simulink library "aausat3_lib"  (Simulink 8.3)
settings: Solver=ode45  StartTime=0.0  StopTime=10.0  RelTol=1e-3
undefined symbols (not defined in the file or in its folder): A_wire_mt, albedo_wrapper, alpha_0_mt, bias_gyro, bias_mag, bias_sun, Cd, coil_dim, Dim, f_sample, G, heading_gyro, heading_mag, M_earth, M_moon, M_sun, magnitude, n_mt, noise_gyro, noise_mag, noise_sun, nr_sample_sun, otoquest, otoquest_with_pro, q_method, qmethod, redfac, refldata, s_freq_gyro, s_freq_mag, s_freq_sun, sigma_0_mt, solar_absorb_coeff, solar_m_flux, SVD_method, T_0_mt, theta_e, tilt_gyro, tilt_mag, Ts
undefined symbols (not defined in the file): Actuator_Duty_Cycle_coil, Actuator_Frequency_coil, Dimensions_coil, mean_refl, Number_of_Windings_coil, rho, sim_par, svd_weigth, Wire_Cross_Sectional_Area_coil, Wire_Resistivity_Base_Temperature_coil, Wire_Resistivity_coil, Wire_Resistivity_Temperature_Coefficient_coil
libraries: aausat3_lib x118, simulink_extras x3
(part 1 of 4)
settings Model: Creator=kasperv  LastModifiedBy=Nemanja

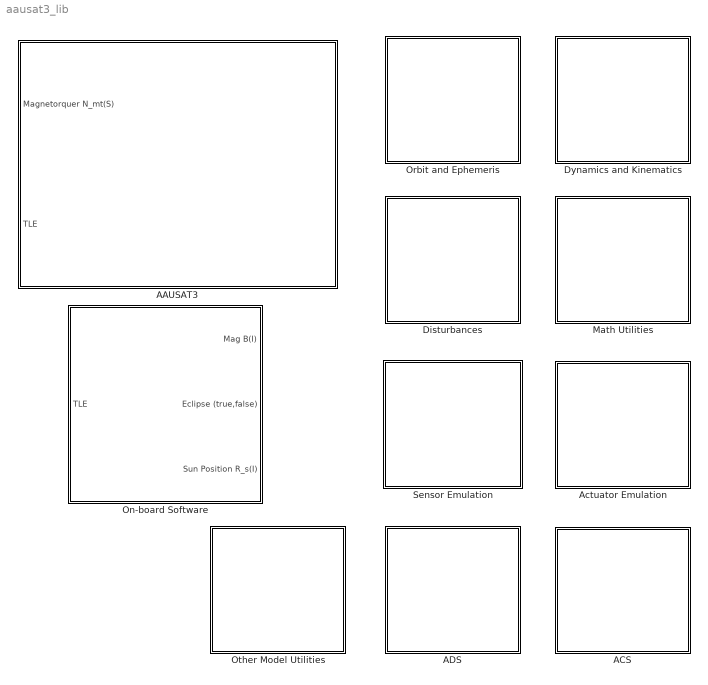
== system aausat3_lib ==
  AAUSAT3 : Subsystem  mask{r_com_s=[0.02 0.001 0.0], sat_temp_start=293.15, mass_sc=2.0, Dim=[0.207 0.1 0.1], inertia_c=[0.007,0.014,0.015], init_jd=2455153.1954318*0, q_s_c=[0 0 0 1], q_init_I_S=[0 1 0 0], w_init_s=[1,1,1]*0.2*(pi/180), Cd=2, rho=0.21850/1e12*0+9.9550/1e12*1+316.2/1e12*0, solar_m_flux=4.5565e-6, solar_absorb_coeff=1.5, theta_e=65, refldata=load('lib/AlbedoToolbox-1.0/refl_data/2005/ga050101-051231'), redfac=1, Ts=1, enable_sensor_emulation=on, enable_env_disturbance=on}
      mask prompts: r_com_s "Center of Mass:"; sat_temp_start "Start Temperature of the Satellite [K]:"; mass_sc "Mass of the Satellite [kg]:"; Dim "Satellite dimension"; inertia_c "Inertia Matrix of the Satellite:"; init_jd "Initial time [JD]:"; q_s_c "Controller Reference Frame (S->C):"; q_init_I_S "Initial Attitude (I->S):"; w_init_s "Initial Angular Rate (S) [rad/s]:"; Cd "Atmospheric Drag Coefficient [-]:"; rho "Atmospheric Density [kg/m^3]:"; solar_m_flux "Solar Momentum Flux [kg/ms^2]:"; solar_absorb_coeff "Solar Absorbtion Coefficient [-]:"; theta_e "Max. Angle of Theta [deg](eclipse: theta>r_earth/norm(R_SA)):"; refldata "Reflectivity Data (REFL Struct):"; redfac "Reduction Factor:"; Ts "Albedo Sampling Time [s]:"; enable_sensor_emulation "Enable Sensor Emulation."; enable_env_disturbance "Enable Environment Disturbance."
      mask Display:
      | image(imread('sat.jpg'));
      | color('w');
      | port_label('input', 1, 'N_mt(S)');
      | port_label('input', 2, 'TLE');
  ACS : Subsystem
      mask Display: image(imread('pictures/control.jpg'))
  ADS : Subsystem
      mask Display: image(imread('pictures/Kalman.jpg'))
  Actuator Emulation : Subsystem
      mask Display: image(imread('pictures/magnetorquer.jpg'))
  Disturbances : Subsystem
      mask Display: image(imread('pictures/noise.jpg'))
  Dynamics and Kinematics : Subsystem
      mask Display: image(imread('pictures/dynamic.jpg'))
  Math Utilities : Subsystem
      mask Display: image(imread('pictures/math.jpg'))
  On-board Software : Subsystem  mask{init_jd=sim_par(20), igrf_order=8, theta_e=65, f_sample=sim_par(22)}
      mask prompts: init_jd "Initial Time [JD]:"; igrf_order "IGRF Model Order [-]:"; theta_e "Max. Angle of Theta [deg]:"; f_sample "Sampling Frequency [Hz]:"
      mask Display:
      | image(imread('pictures/matrix.jpg'));
      | color('w');
      | port_label('input', 1, 'TLE');
      | port_label('output', 1, 'Mag B(I)');
      | port_label('output', 2, 'Eclipse (true,false)');
      | port_label('output', 3, 'Sun Position R_s(I)');
  Orbit and Ephemeris : Subsystem
      mask Display: image(imread('pictures/orbit.jpg'))
  Other Model Utilities : Subsystem
      mask Display: image(imread('pictures/blackboard.jpg'))
  Sensor Emulation : Subsystem
      mask Display: image(imread('pictures/magnetometer.jpg'))

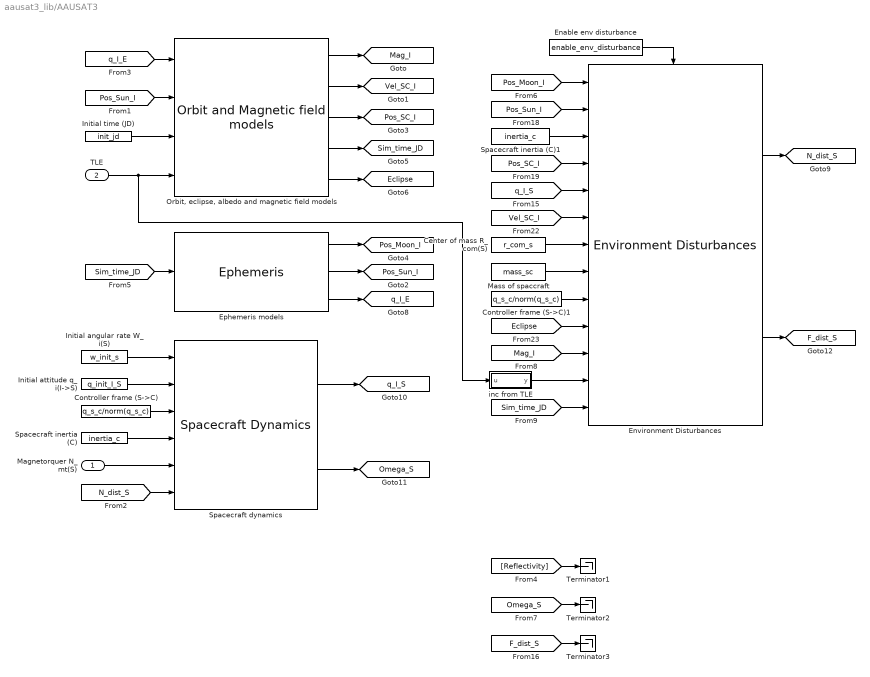
== system aausat3_lib/AAUSAT3 ==
  Magnetorquer N_mt(S) : Inport
  TLE : Inport  Port=2
  Center of mass R_com(S) : Constant  Value=r_com_s
  Controller frame (S->C) : Constant  Value=q_s_c/norm(q_s_c)
  Controller frame (S->C)1 : Constant  Value=q_s_c/norm(q_s_c)
  Enable env disturbance : Constant  Value=enable_env_disturbance
  Environment Disturbances : aausat3_lib/Disturbances/Environment Disturbances  Dim=Dim  sola_m_flux=solar_m_flux  solar_absorb_coeff=solar_absorb_coeff  rho=rho  Cd=Cd  G=6.672e-11  M_sun=1.989e30  M_earth=5.9742e24  M_moon=0.073483e24  enable_rad_dist=on  enable_atmospheric_dist=on  enable_gravity_dist=on  enable_mag_residual_dist=on
  Ephemeris models : aausat3_lib/Orbit and Ephemeris/Ephemeris
  Initial angular rate W_i(S) : Constant  Value=w_init_s
  Initial attitude q_i(I->S) : Constant  Value=q_init_I_S
  Initial time (JD) : Constant  Value=init_jd
  Mass of spaccraft : Constant  Value=mass_sc
  "Orbit, eclipse, albedo and magnetic field models" : aausat3_lib/Orbit and Ephemeris/Orbit and Magnetic field models  theta_e=theta_e  refldata=refldata  redfac=redfac  Ts=Ts  r_e=6371e3  enable_eclipse=on  enable_IGRF=on  reflectivity_enabled=off  enable_sgp4=on  enable_custom_time=on
  Spacecraft dynamics : aausat3_lib/Dynamics and Kinematics/Spacecraft Dynamics
  Spacecraft inertia (C) : Constant  Value=inertia_c
  Spacecraft inertia (C)1 : Constant  Value=inertia_c
  Terminator1 : Terminator
  Terminator2 : Terminator
  Terminator3 : Terminator
  inc from TLE : MATLAB Function  TreatAsAtomicUnit=on
  tag scope: Eclipse=global, F_dist_S=global, Mag_I=global, N_dist_S=global, Omega_S=global, Pos_Moon_I=global, Pos_SC_I=global, Pos_Sun_I=global, Sim_time_JD=global, Vel_SC_I=global, q_I_E=global, q_I_S=global
  wires:
  "Orbit, eclipse, albedo and magnetic field models"/4 -> [Sim_time_JD]
  inc from TLE/1(y) -> Environment Disturbances/12
  [N_dist_S] -> Spacecraft dynamics/6
  [Sim_time_JD] -> Ephemeris models/1
  Spacecraft dynamics/2 -> [Omega_S]
  Ephemeris models/3 -> [q_I_E]
  Ephemeris models/2 -> [Pos_Sun_I]
  Ephemeris models/1 -> [Pos_Moon_I]
  [Sim_time_JD] -> Environment Disturbances/13
  Initial attitude q_i(I->S)/1 -> Spacecraft dynamics/2
  Initial angular rate W_i(S)/1 -> Spacecraft dynamics/1
  "Orbit, eclipse, albedo and magnetic field models"/3 -> [Pos_SC_I]
  Controller frame (S->C)/1 -> Spacecraft dynamics/3
  Spacecraft inertia (C)/1 -> Spacecraft dynamics/4
  "Orbit, eclipse, albedo and magnetic field models"/2 -> [Vel_SC_I]
  "Orbit, eclipse, albedo and magnetic field models"/1 -> [Mag_I]
  Magnetorquer N_mt(S)/1 -> Spacecraft dynamics/5
  "Orbit, eclipse, albedo and magnetic field models"/5 -> [Eclipse]
  [F_dist_S] -> Terminator3/1
  Spacecraft dynamics/1 -> [q_I_S]
  [Pos_Sun_I] -> "Orbit, eclipse, albedo and magnetic field models"/2
  Initial time (JD)/1 -> "Orbit, eclipse, albedo and magnetic field models"/3
  [Reflectivity] -> Terminator1/1
  [Omega_S] -> Terminator2/1
  [q_I_E] -> "Orbit, eclipse, albedo and magnetic field models"/1
  TLE/1 -> "Orbit, eclipse, albedo and magnetic field models"/4, inc from TLE/1(u)
  [Pos_Moon_I] -> Environment Disturbances/1
  Enable env disturbance/1 -> Environment Disturbances/Enable
  [Pos_Sun_I] -> Environment Disturbances/2
  Spacecraft inertia (C)1/1 -> Environment Disturbances/3
  [Pos_SC_I] -> Environment Disturbances/4
  [Vel_SC_I] -> Environment Disturbances/6
  Center of mass R_com(S)/1 -> Environment Disturbances/7
  Mass of spaccraft/1 -> Environment Disturbances/8
  Controller frame (S->C)1/1 -> Environment Disturbances/9
  [Eclipse] -> Environment Disturbances/10
  [Mag_I] -> Environment Disturbances/11
  Environment Disturbances/1 -> [N_dist_S]
  Environment Disturbances/2 -> [F_dist_S]
  [q_I_S] -> Environment Disturbances/5

== system aausat3_lib/ACS ==
  B_dot : Subsystem  mask{C=200000, wc=0.7, m_pm=0.0030, Ts=0.1}
      mask prompts: C "Gain:"; wc "Filter cutoff frequency:"; m_pm "Permanent magnet dipole moment:"; Ts "Sample time:"
  nmpc (AAUSAT3) : Subsystem  mask{f_sample=f_sample}
      mask prompts: f_sample "Sampling Frequency [Hz]"
      mask init:
      | init=0;

== system aausat3_lib/ADS ==
  ADS methods : Subsystem  mask{f_sample=1, svd_weigth=[1/0.0034 1/0.0027], q0_guess=[0 0 1 0], enable_ukf_simple=on, enable_ukf_bias=on, enable_ukf_bias_inertia=off, enable_svd=on}
      mask prompts: f_sample "Sampling Frequency [Hz]:"; svd_weigth "SVD Observations Weights [sun,mag]:"; q0_guess "Initial Attitude Guess [q1,q2,q3,q4]:"; enable_ukf_simple "Enable UKF estimation"; enable_ukf_bias "Enable UKF Plus Bias estimation"; enable_ukf_bias_inertia "Enable UKF Plus Bias and Inertia estimation"; enable_svd "Enable SVD method estimation"
  EKF using quaternions (AAUSAT-II) : Subsystem
  EKF using sun and mag vectors (AAUSAT-II) : Subsystem
  EKF using sun and mag vectors (AAUSAT3) : Subsystem
  EKF using sun and mag vectors ..  and removing bias (AAUSAT-II) : Subsystem
  Propagator from Kalman filter (AAUSAT-II) : Subsystem
  UKF using sun and mag vectors (AAUSAT3) : Subsystem  mask{f_sample=f_sample}
      mask prompts: f_sample "Sampling Frequency [Hz]"
      mask init:
      | init=0;
  UKF using sun and mag vectors .. including bias and inertia estimation (AAUSAT3) : Subsystem  mask{f_sample=f_sample}
      mask prompts: f_sample "Sampling Frequency [Hz]:"
      mask init:
      | init=0;
  UKF using sun and mag vectors .. including bias estimation (AAUSAT3) : Subsystem  mask{f_sample=f_sample}
      mask prompts: f_sample "Sampling Frequency [Hz]:"
      mask init:
      | init=0;
  otoquest (AAUSAT-II) : Subsystem
  otoquest with propagator (AAUSAT-II) : Subsystem
  q-method (AAUSAT-II) : Subsystem
  q-method (AAUSAT3) : Subsystem  mask{weigth_a=[1/(0.031)^2 1/(0.0012)^2]}
      mask prompts: weigth_a "Weigth of the observation vector [-]:"
  svd-method (AAUSAT3) : Subsystem  mask{f_sample=f_sample, weigth_a=svd_weigth}
      mask prompts: f_sample "Sampling Frequency [Hz]:"; weigth_a "Weigth of the Observation Vectors [sun,mag]:"

== system aausat3_lib/Actuator Emulation ==
  Magnetorquer : Subsystem  mask{coil_dim=coil_dim, n_mt=n_mt, A_wire_mt=A_wire_mt, sigma_0_mt=sigma_0_mt, alpha_0_mt=alpha_0_mt, T_0_mt=T_0_mt}
      mask prompts: coil_dim "Coil Dimensions [x,y][m]:"; n_mt "Coil Winding Number [-]:"; A_wire_mt "Wire Cross Sectional Area [m^2]:"; sigma_0_mt "Wire Resistivity [Ohm*m]:"; alpha_0_mt "Wire Resistivity Temperature Coefficient [(deg C)^-1]:"; T_0_mt "Wire Resistivity Base Temperature [K]:"
  Magnetorquers+drivers : Subsystem  mask{coil_dim=Dimensions_coil, n_mt=Number_of_Windings_coil, A_wire_mt=Wire_Cross_Sectional_Area_coil, sigma_0_mt=Wire_Resistivity_coil, alpha_0_mt=Wire_Resistivity_Temperature_Coefficient_coil, T_0_mt=Wire_Resistivity_Base_Temperature_coil, freq_mag=Actuator_Frequency_coil, duty_mag=Actuator_Duty_Cycle_coil}
      mask prompts: coil_dim "Coil Dimensions [x,y][m]:"; n_mt "Coil Winding Number [-]:"; A_wire_mt "Wire Cross Sectional Area [m^2]:"; sigma_0_mt "Wire Resistivity [Ohm*m]:"; alpha_0_mt "Wire Resistivity Temperature Coefficient [(deg C)^-1]:"; T_0_mt "Wire Resistivity Base Temperature [K]:"; freq_mag "Actuator Frequency [Hz]"; duty_mag "Actuator Duty Cycle [%]"
  "Output scaling m -> PWM" : Subsystem  mask{coil_dim=Dimensions_coil, n_mt=Number_of_Windings_coil, A_wire_mt=Wire_Cross_Sectional_Area_coil, sigma_0_mt=Wire_Resistivity_coil, alpha_0_mt=Wire_Resistivity_Temperature_Coefficient_coil, T_0_mt=Wire_Resistivity_Base_Temperature_coil, PWM_max=62.5, PWM_min=37.5}
      mask prompts: coil_dim "Coil Dimensions [x,y][m]:"; n_mt "Coil Winding Number [-]:"; A_wire_mt "Wire Cross Sectional Area [m^2]:"; sigma_0_mt "Wire Resistivity [Ohm*m]:"; alpha_0_mt "Wire Resistivity Temperature Coefficient [(deg C)^-1]:"; T_0_mt "Wire Resistivity Base Temperature [K]:"; PWM_max "PWM max [%]"; PWM_min "PWM min [%]"
  Permanent Magnet : Subsystem  mask{mag_moment=0.0030}
      mask prompts: mag_moment "Magnetic Dipole Moment of the Satellite [Am^2]:"
      mask help: Torque affecting the satellite caused by the magnetic dipole moment.

== system aausat3_lib/Disturbances ==
  Atmospheric : Subsystem  mask{Cd=Cd, rho=rho}
      mask prompts: Cd "Drag Coefficient [-]:"; rho "Atmospheric Density [kg/m^3]:"
      mask help: Force and torque from the atmospheric drag acting on the satellite.
  Environment Disturbances : Subsystem  mask{Dim=Dim, sola_m_flux=solar_m_flux, solar_absorb_coeff=solar_absorb_coeff, rho=rho, Cd=Cd, G=6.672e-11, M_sun=1.989e30, M_earth=5.9742e24, M_moon=0.073483e24, enable_rad_dist=on, enable_atmospheric_dist=on, enable_gravity_dist=on, enable_mag_residual_dist=on}
      mask prompts: Dim "Satellite Dimension [x,y,z][m]:"; sola_m_flux "Solar Momentum Flux [kg/ms^2]:"; solar_absorb_coeff "Solar Absorbtion Coefficient [-]:"; rho "Atmospheric Density [kg/m^3]:"; Cd "Atmospheric Drag Coefficient [-]:"; G "Gravitational Constant [m^3/kgs^2]:"; M_sun "Mass of the Sun [kg]:"; M_earth "Mass of the Earth [kg]:"; M_moon "Mass of the Moon [kg]:"; enable_rad_dist "Enable Radiation Disturbanceses."; enable_atmospheric_dist "Enable Atmospheric Disturbanceses."; enable_gravity_dist "Enable Gravity Disturbanceses."; enable_mag_residual_dist "Enable Magnetic Residual Disturbance"
      mask help: Torque and force from the environment affecting the satellite.
  Gravity : Subsystem  mask{G=G, M_sun=M_sun, M_moon=M_moon, M_earth=M_earth, enable_moon_G=on, enable_sun_G=on, enable_zharm_earth=on, enable_gravity_torque=on}
      mask prompts: G "Gravitational Constant [m^3/kgs^2]:"; M_sun "Mass of the Sun [kg]:"; M_moon "Mass of the Moon [kg]:"; M_earth "Mass of the Earth [kg]:"; enable_moon_G "Enable the Gravity of the Moon."; enable_sun_G "Enable the Gravity of the Sun."; enable_zharm_earth "Enable the Earth Zonal Harmonics."; enable_gravity_torque "Enable Torque From Gravity."
  Gravity Gradient Torque : Subsystem  mask{G=G, M_earth=M_earth}
      mask prompts: G "Gravitational Constant [m^3/kgs^2]:"; M_earth "Mass of the Earth [kg]:"
      mask help: Gravitational force applied by the Earth.
  Gravity Moon : Subsystem  mask{G=G, M_moon=M_moon}
      mask prompts: G "Gravitational Constant [m^3/kgs^2]:"; M_moon "Mass of the Moon [kg]:"
      mask help: Gravitational force applied by the Moon.
  Gravity Sun : Subsystem  mask{G=G, M_sun=M_sun}
      mask prompts: G "Gravitational Constant [m^3/kgs^2]:"; M_sun "Mass of the Sun [kg]:"
      mask help: Gravitational force applied by the Sun.
  Magnetic Residual Disturbance : Subsystem  mask{mag_moment=0.00033}
      mask prompts: mag_moment "Magnetic Dipole Moment of the Satellite [Am^2]:"
      mask help: Torque affecting the satellite caused by the magnetic dipole moment.
  Radiation (I) : Subsystem  mask{Dim=Dim, solar_m_flux=solar_m_flux, solar_absorb_coeff=solar_absorb_coeff}
      mask prompts: Dim "Satellite Dimension [x,y,z][m]:"; solar_m_flux "Solar Momentum Flux [kg/ms^2]:"; solar_absorb_coeff "Absorbtion Coefficient [-]:"
      mask help: Solar force and torque acting on the satellite.
  Zonal Harmonics  Earth : Subsystem

== system aausat3_lib/Dynamics and Kinematics ==
  Spacecraft Dynamics : Subsystem

== system aausat3_lib/Math Utilities ==
  Projection Matrix : Subsystem
  Quaternion operations : Subsystem
  Rotation matrix  to quaternion : MATLABFcn  Description=|  MATLABFcn=A_to_q
      | Converts a rotation matrix to a quaternion.                
      |                                                            
      | The implementation is implemented to be numerically robust.
  Vector operations : Subsystem
  q_i_o calculator : Subsystem

== system aausat3_lib/On-board Software ==
  TLE : Inport
  Constant : Constant  Value=init_jd  SampleTime=1/f_sample
  Ephemeris : Subsystem
  Orbit and Magnetic field models : Subsystem  mask{r_e=6371e3, theta_e=theta_e, init_jd=init_jd, igrf_order=igrf_order, enable_eclipse=on, enable_IGRF=on, enable_sgp4=on, enable_custom_time=on}
      mask prompts: r_e "Radius of the Earth [m]:"; theta_e "Max. Angle of Theta [deg] (eclipse: theta > r_earth/norm(R_SA)):"; init_jd "Initial Time [JD]:"; igrf_order "IGRF Model Order [-]:"; enable_eclipse "Enable Eclipse Model."; enable_IGRF "Enable IGRF Model."; enable_sgp4 "Enable SGP4 Model."; enable_custom_time "Enable Custom Time."
  Mag B(I) : Outport  SampleTime=1/f_sample
  Eclipse (true,false) : Outport  Port=2  SampleTime=1/f_sample
  Sun Position R_s(I) : Outport  Port=3  SampleTime=1/f_sample
  tag scope: Sim_time_JD_sat=global, q_I_E_sat=global
  wires:
  Orbit and Magnetic field models/2(Simulation time t(JD)) -> [Sim_time_JD_sat]
  Orbit and Magnetic field models/3("Eclipse: 1=true, 0=false") -> Eclipse (true,false)/1
  Orbit and Magnetic field models/1(Mag [Tesla] B(I)) -> Mag B(I)/1
  TLE/1 -> Orbit and Magnetic field models/4(TLE)
  [Sim_time_JD_sat] -> Ephemeris/1(Time t(JD))
  [q_I_E_sat] -> Orbit and Magnetic field models/1(Earth rotation q(I->E))
  Ephemeris/1(Sun Position R_s(I)) -> Sun Position R_s(I)/1, Orbit and Magnetic field models/2(Sun position R_s(I))
  Ephemeris/2(Earth Rotation q(I->E)) -> [q_I_E_sat]
  Constant/1 -> Orbit and Magnetic field models/3(Initial time ti(JD))

== system aausat3_lib/Orbit and Ephemeris ==
  (IGRF) Magnetic field : Subsystem  TreatAsAtomicUnit=on
  Albedo : Subsystem  TreatAsAtomicUnit=on  mask{refldata=mean_refl, redfac=1, Ts=-1}
      mask prompts: refldata "Reflectivity Data (REFL Struct):"; redfac "Reduction factor:"; Ts "Sample Time (-1 for inherited):"
  Custom time : Subsystem  TreatAsAtomicUnit=on
  ECI->ECEF quaternion : Subsystem
  Eclipse model : Subsystem  mask{r_e=6371000, enable=off, theta_e=65}
      mask prompts: r_e "Radius of Earth [m]"; enable "Enable max angle"; theta_e "Max. angle of theta [deg] (eclipse: theta > r_earth/norm(R_SA))"
      mask Display: fprintf('1=true,\n 0=false')
  Ephemeris : Subsystem
  Magnetic field model : Subsystem
  Orbit and Magnetic field models : Subsystem  mask{theta_e=theta_e, refldata=refldata, redfac=redfac, Ts=Ts, r_e=6371e3, enable_eclipse=on, enable_IGRF=on, reflectivity_enabled=off, enable_sgp4=on, enable_custom_time=on}
      mask prompts: theta_e "Max. Angle of Theta [deg] (eclipse: theta > r_earth/norm(R_SA)):"; refldata "Reflectivity Data (REFL Struct):"; redfac "Reduction Factor:"; Ts "Albedo Model Sampling Time [s]:"; r_e "Radius of the Earth [m]:"; enable_eclipse "Enable Eclipse Model."; enable_IGRF "Enable IGRF Model."; reflectivity_enabled "Enable Albedo Model."; enable_sgp4 "Enable SGP4 Model."; enable_custom_time "Enable Custom Time."
      mask help: When you want to use "Other" make sure to define the TLE in the SGP4 subsystem.
  SGP4 position : Subsystem  TreatAsAtomicUnit=on
  TLE AAUSAT-II : Subsystem  mask{satname='AAUSAT-II', JulianDay=09279.82913737, xndt2o=0.00000416, xndd6o=0.0, bstar=.59418e-4, xincl=97.9326, xnodeo=342.7215, eo=0.0016322, omegao=34.9001, xmo=325.3249, xno=14.81792083, ts=1}
      mask prompts: satname "Satellite Name:"; JulianDay "Epoch [YYDDD.DDDDDDDD]:"; xndt2o "Mean Motion 1st [rev/day^2]:"; xndd6o "Mean Motion 2nd [rev/day^3]:"; bstar "B* Drag [Earth radii^-1]"; xincl "Inclination [deg]:"; xnodeo "Right Ascension of Ascending Node [deg]:"; eo "Eccentricity [-]:"; omegao "Argument of Perigee [deg]:"; xmo "Mean Anomaly [deg]:"; xno "Mean Motion [rev/day]:"; ts "Sampling Time [sec]:"
      mask help: Two-Line Orbital Element Set Format.
      mask Display: fprintf('TLE Object \n Satellite Name: %s\n Epoch: %d',satname,floor(JulianDay));
  TLE AAUSAT-II (2) : aausat3_lib/Orbit and Ephemeris/TLE AAUSAT-II  satname='AAUSAT-II'  JulianDay=09321.69542252  xndt2o=0.00000555  xndd6o=0.0  bstar=.76898e-4  xincl=97.9251  xnodeo=24.1597  eo=0.0014245  omegao=254.1774  xmo=105.7862  xno=14.81823818  ts=1
  TLE Orsted : Subsystem  mask{satname='Orsted', YYDDD=02039, JulianDay=2452275.5+40.69255057, xndt2o=0.00002748*0, xndd6o=0, bstar=0.00071190, xincl=96.4788, xnodeo=112.1945, eo=0.0148615, omegao=71.6037, xmo=290.1241, xno=14.43891950, ts=1}
      mask prompts: satname "Satellite Name:"; YYDDD "Epoch [YYDDD]:"; JulianDay "Epoch [JD]:"; xndt2o "Mean Motion 1st [rev/day^2]:"; xndd6o "Mean Motion 2nd [rev/day^3]:"; bstar "B* Drag [Earth radii^-1]"; xincl "Inclination [deg]:"; xnodeo "Right Ascension of Ascending Node [deg]:"; eo "Eccentricity [-]:"; omegao "Argument of Perigee [deg]:"; xmo "Mean Anomaly [deg]:"; xno "Mean Motion [rev/day]:"; ts "Sampling Time [sec]:"
      mask help: Two-Line Orbital Element Set Format.
      mask Display: fprintf('TLE Object \n Satellite Name: %s\n Epoch: %d',satname,YYDDD);

== system aausat3_lib/Other Model Utilities ==
  AAUSAT-II Animation : Subsystem  mask(AAUSAT-II Animation){u1=[-20000000 20000000 -20000000 20000000 -20000000 20000000], u2=1, u3=300000, u20=on, u18=15, u4=6378000, u11=150, u12=on, u13='earth3150.jpg', u17=180, u5=Fixed position, u6=[70000000 70000000 70000000], u7=8, u9=off, u10=on, u16=off, u14=on, u15=on, u8=on, u19=off}
      mask prompts: u1 "Axes limits [xmin xmax ymin ymax zmin zmax]:"; u2 "Time interval between updates:"; u3 "Size of spacecraft displayed:"; u20 "Use spacecraft image map"; u18 "Spacecraft drawing slices"; u4 "Planet radius:"; u11 "Planet drawing slices"; u12 "Use planet map"; u13 "Planet map image file"; u17 "Pre-rotate image map (deg)"; u5 "Enter view:"; u6 "Position of camera [xc yc zc]:"; u7 "View angle:"; u9 "Show SC coordinate system"; u10 "Show orbit coordinate system"; u16 "Show Earth Centered Earth Fixed coordinate system"; u14 "Show inertial coordinate system"; u15 "Show trajectory"; u8 "Enable animation"; u19 "Make movie (use with care!)"
      mask help:
      | Create a 3-D animated view of the AAUSAT-II, where X, Y, and Z craft position (Position) and craft quaternion (Attitude) are inputs.
      |
      | Display parameters are in the same units of length as the input parameters.
      |
      | Created by Karl Laursen
      mask init:
      | Config.axes = u1;
      | Config.update = u2;
      | Config.craft = u3;
      | Config.radius = u4;
      | Config.camera_view = u5;
      | Config.camera_pos = u6;
      | Config.view = u7;
      | Config.Animenable = u8;
      | Config.ShowSCFrame = u9;
      | Config.ShowOrbitFrame = u10;
      | Config.ShowECEF = u16;
      | Config.ShowInertial = u14;
      | Config.PlanetSlices = u11;
      | Config.UseMap = u12;
      | Config.PlanetMapFile = u13;
      | Config.Trajectory = u15;
      | Config.PreRotation = u17;
      | Config.CraftSlices = u18;
      | Config.MakeMovie = u19;
      | Config.UseSCMap = u20;
      mask Help: web(asbhelp('6dofanimation'));
      mask TypeOptions u5: Fixed position | Fly alongside
  Exposed area : Subsystem  mask{dim_sat_area=[0.1,0.2,0.1]}
      mask prompts: dim_sat_area "Satellite Dimentions [x,y,z] [m]:"
      mask help: Calculates the exposed area of the satellite.
  Geocentric to  Geodetic Latitude : Subsystem  mask(Geocentric to Geodetic Latitude){F=, R=}
      mask prompts: F "Flattening:"; R "Equatorial radius of planet:"
      mask help: Convert geocentric latitude to geodetic latitude. Geodetic latitude is computed using geocentric latitude and the radius from the center of the planet to the center of gravity.
      mask init:
      | F=1/298.257223563;
      | R=6378137;
      mask Help: eval('asbhelp');
      mask Display:
      | port_label('input',1,'\lambda','texmode','on')
      | port_label('input',2,'r','texmode','on')
      | port_label('output',1,'\mu','texmode','on')
  Geodetic to  Geocentric Latitude : Subsystem  mask(Geodetic to Geocentric Latitude){F=1/298.257223563, R=6378137}
      mask prompts: F "Flattening:"; R "Equatorial radius of planet:"
      mask help: Convert geodetic latitude to geocentric latitude. Setting mean sea-level altitude to zero will give the geocentric latitude at the surface of the planet.
      mask Help: eval('asbhelp');
      mask Display:
      | port_label('input',1,'\mu','texmode','on')
      | port_label('input',2,'h','texmode','on')
      | port_label('output',1,'\lambda','texmode','on')
  Randome 3D Vector : Subsystem  mask{mean=0, var=100, seed=[23314,67594,99812]}
      mask prompts: var "Variance:"; seed "Seed [s1,s2,s3]:"
  SC ECI to geodetic position converter : Subsystem
      mask help:
      | Converts the spacecraft position in the ECI frame to geodetic coordinates.
      | Can be used to plot spacecraft position on a world map.
      mask init:
      | a=6378.1370;
      | b=6356.7523;
  Satellite Area : Subsystem
  Store data : Subsystem  mask{f_sample=1, enable_t=on, enable_att=on, enable_w=on, enable_att_ukf=on, enable_w_ukf=on, enable_r_sun=on, enable_r_mag=on, enable_r_w=on, enable_eia=on, enable_eiw=on, enable_att_ukf_bias=on, enable_w_ukf_bias=on, enable_b_mag=on, enable_b_gyro=on, enable_r_sun_ukf_bias=on, enable_r_mag_ukf_bias=on, enable_r_w_ukf_bias=on, enable_eia_ukf_bias=on, enable_eiw_ukf_bias=on, enable_att_svd=on, enable_svd_att_err=on, enable_svd_err=on, enable_tictoc=on, enable_tictoc_ukf_bias=on, enable_tictoc_svd=on, enable_n_dist=on, enable_n_pmag=on, enable_n_con=on, enable_eclip_sw=on, enable_eclip_real=on}
      mask prompts: f_sample "Sampling Frequency [Hz]:"; enable_t "Store Time"; enable_att "Store Real Attitude"; enable_w "Store Real Angular Velocity"; enable_att_ukf "Store Estimated Attitude (UKF)"; enable_w_ukf "Store Estimated Angular Velocity (UKF)"; enable_r_sun "Store Sun Vector Residual (UKF)"; enable_r_mag "Store Magnetic Field Vector Residual (UKF)"; enable_r_w "Store Angular Velocity Residual (UKF)"; enable_eia "Store Error in Attitude  (UKF)"; enable_eiw "Store Error in Angular Velocity (UKF)"; enable_att_ukf_bias "Store Estimated Attitude (UKF Bias)"; enable_w_ukf_bias "Store Estimated Angular Velocity (UKF Bias)"; enable_b_mag "Store Magnetometer Bias (UKF Bias)"; enable_b_gyro "Store Gyro Bias (UKF Bias)"; enable_r_sun_ukf_bias "Store Sun Vector Residual (UKF Bias)"; enable_r_mag_ukf_bias "Store Magnetic Field Vector Residual (UKF Bias)"; enable_r_w_ukf_bias "Store Angular Velocity Residual (UKF Bias)"; enable_eia_ukf_bias "Store Error in Attitude  (UKF Bias)"; enable_eiw_ukf_bias "Store Error in Angular Velocity (UKF Bias)"; enable_att_svd "Store Estimated Attitude (SVD)"; enable_svd_att_err "Store Error in Attitude (SVD)"; enable_svd_err "Store SVD Error Indicator"; enable_tictoc "Store Algorithm Execution Time (UKF)"; enable_tictoc_ukf_bias "Store Algorithm Execution Time (UKF Bias)"; enable_tictoc_svd "Store Algorithm Execution Time (SVD)"; enable_n_dist "Store Environment Disturbances"; enable_n_pmag "Store Permanent Magnet Disturbance"; enable_n_con "Store Control Torque"; enable_eclip_sw "Stor On-board Software Eclipse Indicator"; enable_eclip_real "Store the Real Eclipse Indicator"
  "TLE -> JD converter" : Subsystem

== system aausat3_lib/Sensor Emulation ==
  Gyroscopes : Subsystem  mask{s_freq_gyro=s_freq_gyro, noise_gyro=noise_gyro, bias_gyro=bias_gyro, heading_gyro=heading_gyro, tilt_gyro=tilt_gyro}
      mask prompts: s_freq_gyro "Sampling Frequency [Hz]:"; noise_gyro "Noise [deg/s]:"; bias_gyro "Bias (x,y,z) [deg/s]:"; heading_gyro "Sensor placement error (heading) [deg]:"; tilt_gyro "Sensor placement error (tilt) [deg]:"
  Magnetometers : Subsystem  mask{s_freq_mag=s_freq_mag, noise_mag=noise_mag, bias_mag=bias_mag, heading_mag=heading_mag, tilt_mag=tilt_mag}
      mask prompts: s_freq_mag "Sampling Frequency [Hz]:"; noise_mag "Noise [deg]:"; bias_mag "Bias (x,y,z) [nT]:"; heading_mag "Sensor placement error (heading) [deg]:"; tilt_mag "Sensor placement error (tilt) [deg]:"
  Measurements : Subsystem  mask{s_freq_mag=1, noise_mag=3, bias_mag=[0 0 0], heading_mag=0, tilt_mag=0, s_freq_sun=1, noise_sun=3.33, bias_sun=[0 0], nr_sample_sun=1, s_freq_gyro=1, noise_gyro=0.2, bias_gyro=[0 0 0], heading_gyro=0, tilt_gyro=0}
      mask prompts: s_freq_mag "Magnetometer Sampling Frequency [Hz]:"; noise_mag "Magnetometer Noise [deg]:"; bias_mag "Magnetometer Bias (x,y,z) [nT]:"; heading_mag "Magnetometer Placement Error (heading) [deg]:"; tilt_mag "Magnetometer Placement Error (tilt) [deg]:"; s_freq_sun "Sun Sensor Sampling Frequency [Hz]:"; noise_sun "Sun Sensor Noise [deg]:"; bias_sun "Sun Sensor Bias (theta,phi) [deg]:"; nr_sample_sun "Number of Sun Samples [-]:"; s_freq_gyro "Gyroscope Sampling Frequency [Hz]:"; noise_gyro "Gyroscope Noise [deg/s]:"; bias_gyro "Gyroscope Bias (x,y,z) [deg/s]:"; heading_gyro "Gyroscope Placement Error (heading) [deg]:"; tilt_gyro "Gyroscope Placement Error (tilt) [deg]:"
  Sun sensors : Subsystem  mask{s_freq_sun=s_freq_sun, noise_sun=noise_sun, bias_sun=bias_sun, nr_sample_sun=nr_sample_sun}
      mask prompts: s_freq_sun "Sampling Frequency [Hz]:"; noise_sun "Noise [deg]:"; bias_sun "Bias (theta,phi) [deg]:"; nr_sample_sun "Number of Samples [-]:"

== system aausat3_lib/ACS/B_dot ==
  B_meas : Inport
  Gain : Gain  Gain=-C
  Gain1 : Gain  Gain=wc
  Gain2 : Gain  Gain=exp(-wc*Ts)
  Permanent magnet  dipole moment : Constant  Value=[0,0,m_pm]
  Sum2 : Sum  Inputs=-++
  Sum3 : Sum  Inputs=|++
  Unit Delay : UnitDelay  SampleTime=-1
  Unit Delay1 : UnitDelay  SampleTime=-1
  m_ctrl : Outport  PortDimensions=3
  wires:
  B_meas/1 -> Gain1/1
  Unit Delay/1 -> Sum2/1
  Gain1/1 -> Unit Delay/1, Sum2/2
  Gain2/1 -> Sum2/3
  Unit Delay1/1 -> Gain2/1
  Sum2/1 -> Unit Delay1/1, Gain/1
  Permanent magnet  dipole moment/1 -> Sum3/2
  Gain/1 -> Sum3/1
  Sum3/1 -> m_ctrl/1

== system aausat3_lib/ACS/nmpc (AAUSAT3) ==
  x0 : Inport
  q_ref : Inport  Port=2
  simtime_JD : Inport  Port=3
  Enable : EnablePort
  Mux2 : Mux  Inputs=3
  UKF : MATLABFcn  MATLABFcn=nmpc  OutputDimensions=3  SampleTime=1/f_sample
  Uctrl : Outport
  wires:
  q_ref/1 -> Mux2/2
  x0/1 -> Mux2/1
  UKF/1 -> Uctrl/1
  Mux2/1 -> UKF/1
  simtime_JD/1 -> Mux2/3

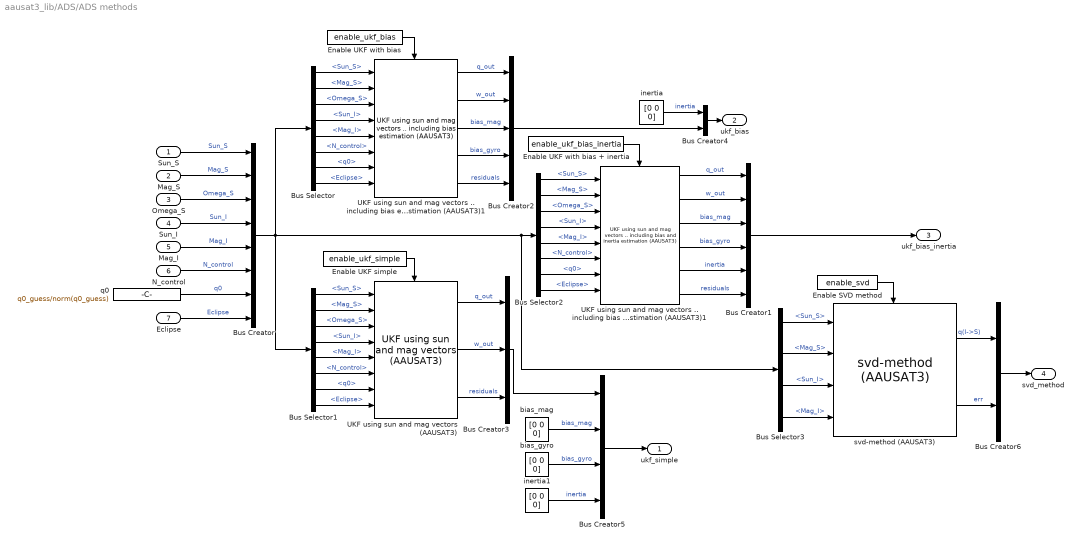
== system aausat3_lib/ADS/ADS methods ==
  Sun_S : Inport
  Mag_S : Inport  Port=2
  Omega_S : Inport  Port=3
  Sun_I : Inport  Port=4
  Mag_I : Inport  Port=5
  N_control : Inport  Port=6
  Eclipse : Inport  Port=7
  Bus Creator : BusCreator  Inputs=8
  Bus Creator1 : BusCreator  Inputs=6
  Bus Creator2 : BusCreator  Inputs=5
  Bus Creator3 : BusCreator  Inputs=3
  Bus Creator4 : BusCreator  Inputs=2
  Bus Creator5 : BusCreator
  Bus Creator6 : BusCreator  Inputs=2
  Bus Selector : BusSelector  OutputSignals=Sun_S,Mag_S,Omega_S,Sun_I,Mag_I,N_control,q0,Eclipse
  Bus Selector1 : BusSelector  OutputSignals=Sun_S,Mag_S,Omega_S,Sun_I,Mag_I,N_control,q0,Eclipse
  Bus Selector2 : BusSelector  OutputSignals=Sun_S,Mag_S,Omega_S,Sun_I,Mag_I,N_control,q0,Eclipse
  Bus Selector3 : BusSelector  OutputSignals=Sun_S,Mag_S,Sun_I,Mag_I
  Enable SVD method : Constant  Value=enable_svd
  Enable UKF simple : Constant  Value=enable_ukf_simple
  Enable UKF with bias : Constant  Value=enable_ukf_bias
  Enable UKF with bias + inertia : Constant  Value=enable_ukf_bias_inertia
  UKF using sun and mag vectors (AAUSAT3) : aausat3_lib/ADS/UKF using sun and mag vectors (AAUSAT3)  SystemSampleTime=-1  f_sample=f_sample
  UKF using sun and mag vectors .. including bias and inertia estimation (AAUSAT3)1 : aausat3_lib/ADS/UKF using sun and mag vectors .. including bias and inertia estimation (AAUSAT3)  SystemSampleTime=-1  f_sample=f_sample
  UKF using sun and mag vectors .. including bias estimation (AAUSAT3)1 : aausat3_lib/ADS/UKF using sun and mag vectors .. including bias estimation (AAUSAT3)  SystemSampleTime=-1  f_sample=f_sample
  bias_gyro : Constant  Value=[0 0 0]
  bias_mag : Constant  Value=[0 0 0]
  inertia : Constant  Value=[0 0 0]
  inertia1 : Constant  Value=[0 0 0]
  q0 : Constant  Value=q0_guess/norm(q0_guess)
  svd-method (AAUSAT3) : aausat3_lib/ADS/svd-method (AAUSAT3)  SystemSampleTime=-1  f_sample=f_sample  weigth_a=svd_weigth
  ukf_simple : Outport
  ukf_bias : Outport  Port=2
  ukf_bias_inertia : Outport  Port=3
  svd_method : Outport  Port=4
  wires:
  Bus Creator6/1 -> svd_method/1
  svd-method (AAUSAT3)/2 -> Bus Creator6/2  "err"
  svd-method (AAUSAT3)/1 -> Bus Creator6/1  "q(I->S)"
  Bus Creator/1 -> Bus Selector/1, Bus Selector1/1, Bus Selector3/1, Bus Selector2/1
  Bus Creator5/1 -> ukf_simple/1
  inertia1/1 -> Bus Creator5/4  "inertia"
  bias_gyro/1 -> Bus Creator5/3  "bias_gyro"
  bias_mag/1 -> Bus Creator5/2  "bias_mag"
  Bus Creator3/1 -> Bus Creator5/1
  Bus Creator4/1 -> ukf_bias/1
  Bus Creator2/1 -> Bus Creator4/2
  inertia/1 -> Bus Creator4/1  "inertia"
  Sun_S/1 -> Bus Creator/1  "Sun_S"
  Mag_S/1 -> Bus Creator/2  "Mag_S"
  Omega_S/1 -> Bus Creator/3  "Omega_S"
  Sun_I/1 -> Bus Creator/4  "Sun_I"
  Mag_I/1 -> Bus Creator/5  "Mag_I"
  N_control/1 -> Bus Creator/6  "N_control"
  q0/1 -> Bus Creator/7  "q0"
  Eclipse/1 -> Bus Creator/8  "Eclipse"
  Bus Selector/1 -> UKF using sun and mag vectors .. including bias estimation (AAUSAT3)1/1  "<Sun_S>"
  Bus Selector/2 -> UKF using sun and mag vectors .. including bias estimation (AAUSAT3)1/2  "<Mag_S>"
  Bus Selector/3 -> UKF using sun and mag vectors .. including bias estimation (AAUSAT3)1/3  "<Omega_S>"
  Bus Selector/4 -> UKF using sun and mag vectors .. including bias estimation (AAUSAT3)1/4  "<Sun_I>"
  Bus Selector/5 -> UKF using sun and mag vectors .. including bias estimation (AAUSAT3)1/5  "<Mag_I>"
  Bus Selector/6 -> UKF using sun and mag vectors .. including bias estimation (AAUSAT3)1/6  "<N_control>"
  Bus Selector/7 -> UKF using sun and mag vectors .. including bias estimation (AAUSAT3)1/7  "<q0>"
  Bus Selector/8 -> UKF using sun and mag vectors .. including bias estimation (AAUSAT3)1/8  "<Eclipse>"
  Enable UKF with bias/1 -> UKF using sun and mag vectors .. including bias estimation (AAUSAT3)1/Enable
  Enable UKF simple/1 -> UKF using sun and mag vectors (AAUSAT3)/Enable
  Enable UKF with bias + inertia/1 -> UKF using sun and mag vectors .. including bias and inertia estimation (AAUSAT3)1/Enable
  Bus Selector1/1 -> UKF using sun and mag vectors (AAUSAT3)/1  "<Sun_S>"
  Bus Selector1/2 -> UKF using sun and mag vectors (AAUSAT3)/2  "<Mag_S>"
  Bus Selector1/3 -> UKF using sun and mag vectors (AAUSAT3)/3  "<Omega_S>"
  Bus Selector1/4 -> UKF using sun and mag vectors (AAUSAT3)/4  "<Sun_I>"
  Bus Selector1/5 -> UKF using sun and mag vectors (AAUSAT3)/5  "<Mag_I>"
  Bus Selector1/6 -> UKF using sun and mag vectors (AAUSAT3)/6  "<N_control>"
  Bus Selector1/7 -> UKF using sun and mag vectors (AAUSAT3)/7  "<q0>"
  Bus Selector1/8 -> UKF using sun and mag vectors (AAUSAT3)/8  "<Eclipse>"
  Bus Selector2/1 -> UKF using sun and mag vectors .. including bias and inertia estimation (AAUSAT3)1/1  "<Sun_S>"
  Bus Selector2/2 -> UKF using sun and mag vectors .. including bias and inertia estimation (AAUSAT3)1/2  "<Mag_S>"
  Bus Selector2/3 -> UKF using sun and mag vectors .. including bias and inertia estimation (AAUSAT3)1/3  "<Omega_S>"
  Bus Selector2/4 -> UKF using sun and mag vectors .. including bias and inertia estimation (AAUSAT3)1/4  "<Sun_I>"
  Bus Selector2/5 -> UKF using sun and mag vectors .. including bias and inertia estimation (AAUSAT3)1/5  "<Mag_I>"
  Bus Selector2/6 -> UKF using sun and mag vectors .. including bias and inertia estimation (AAUSAT3)1/6  "<N_control>"
  Bus Selector2/7 -> UKF using sun and mag vectors .. including bias and inertia estimation (AAUSAT3)1/7  "<q0>"
  Bus Selector2/8 -> UKF using sun and mag vectors .. including bias and inertia estimation (AAUSAT3)1/8  "<Eclipse>"
  Bus Selector3/1 -> svd-method (AAUSAT3)/1  "<Sun_S>"
  Bus Selector3/2 -> svd-method (AAUSAT3)/2  "<Mag_S>"
  Bus Selector3/3 -> svd-method (AAUSAT3)/3  "<Sun_I>"
  Bus Selector3/4 -> svd-method (AAUSAT3)/4  "<Mag_I>"
  Enable SVD method/1 -> svd-method (AAUSAT3)/Enable
  UKF using sun and mag vectors .. including bias and inertia estimation (AAUSAT3)1/1 -> Bus Creator1/1  "q_out"
  UKF using sun and mag vectors .. including bias and inertia estimation (AAUSAT3)1/2 -> Bus Creator1/2  "w_out"
  UKF using sun and mag vectors .. including bias and inertia estimation (AAUSAT3)1/3 -> Bus Creator1/3  "bias_mag"
  UKF using sun and mag vectors .. including bias and inertia estimation (AAUSAT3)1/4 -> Bus Creator1/4  "bias_gyro"
  UKF using sun and mag vectors .. including bias and inertia estimation (AAUSAT3)1/5 -> Bus Creator1/5  "inertia"
  UKF using sun and mag vectors .. including bias and inertia estimation (AAUSAT3)1/6 -> Bus Creator1/6  "residuals"
  UKF using sun and mag vectors .. including bias estimation (AAUSAT3)1/1 -> Bus Creator2/1  "q_out"
  UKF using sun and mag vectors .. including bias estimation (AAUSAT3)1/2 -> Bus Creator2/2  "w_out"
  UKF using sun and mag vectors .. including bias estimation (AAUSAT3)1/3 -> Bus Creator2/3  "bias_mag"
  UKF using sun and mag vectors .. including bias estimation (AAUSAT3)1/4 -> Bus Creator2/4  "bias_gyro"
  UKF using sun and mag vectors .. including bias estimation (AAUSAT3)1/5 -> Bus Creator2/5  "residuals"
  Bus Creator1/1 -> ukf_bias_inertia/1
  UKF using sun and mag vectors (AAUSAT3)/1 -> Bus Creator3/1  "q_out"
  UKF using sun and mag vectors (AAUSAT3)/2 -> Bus Creator3/2  "w_out"
  UKF using sun and mag vectors (AAUSAT3)/3 -> Bus Creator3/3  "residuals"

== system aausat3_lib/ADS/EKF using quaternions (AAUSAT-II) ==
  q : Inport
  w : Inport  Port=2
  h_mw : Inport  Port=3
  N_mt : Inport  Port=4
  q0_in : Inport  Port=5
  eclipse : Inport  Port=6
  Clock : Clock
  Demux1 : Demux  Outputs=16
  EKF : MATLABFcn  MATLABFcn=AAUSAT_II_Kalman  OutputDimensions=16  SampleTime=0.1
  Mux1 : Mux  Inputs=3
  Mux2 : Mux  Inputs=8
  Mux3 : Mux
  Mux4 : Mux  Inputs=3
  Mux5 : Mux  Inputs=3
  Step size : Constant  Value=0.1
  q_out : Outport
  w_out : Outport  Port=2
  q_residual : Outport  Port=3
  w_residual : Outport  Port=4
  wires:
  Demux1/13 -> Mux5/3
  Demux1/12 -> Mux5/2
  Demux1/11 -> Mux5/1
  Demux1/7 -> Mux4/3
  Demux1/6 -> Mux4/2
  Demux1/5 -> Mux4/1
  Demux1/10 -> Mux1/3
  Demux1/9 -> Mux1/2
  Demux1/8 -> Mux1/1
  Mux5/1 -> w_residual/1
  Mux1/1 -> q_residual/1
  Mux2/1 -> EKF/1
  EKF/1 -> Demux1/1
  Step size/1 -> Mux2/7
  Demux1/1 -> Mux3/1
  Demux1/2 -> Mux3/2
  Demux1/3 -> Mux3/3
  Demux1/4 -> Mux3/4
  Clock/1 -> Mux2/5
  w/1 -> Mux2/2
  h_mw/1 -> Mux2/3
  N_mt/1 -> Mux2/4
  Mux3/1 -> q_out/1
  Mux4/1 -> w_out/1
  q/1 -> Mux2/1
  q0_in/1 -> Mux2/6
  eclipse/1 -> Mux2/8

== system aausat3_lib/ADS/EKF using sun and mag vectors (AAUSAT-II) ==
  R_sun(S) : Inport
  b(S) : Inport  Port=2
  w(S) : Inport  Port=3
  R_sun(I) : Inport  Port=4
  b(I) : Inport  Port=5
  h_mw : Inport  Port=6
  N_mt : Inport  Port=7
  q0 : Inport  Port=8
  Eclipse : Inport  Port=9
  Clock : Clock
  Demux1 : Demux  Outputs=7
  EKF : MATLABFcn  MATLABFcn=AAUSAT_II_Kalman_BS_vectors  OutputDimensions=7  SampleTime=0.1
  Mux2 : Mux  Inputs=11
  Mux3 : Mux
  Mux4 : Mux  Inputs=3
  Step size : Constant  Value=0.1
  q_out : Outport
  w_out : Outport  Port=2
  wires:
  w(S)/1 -> Mux2/3
  Eclipse/1 -> Mux2/11
  Demux1/1 -> Mux3/1
  Demux1/2 -> Mux3/2
  Demux1/3 -> Mux3/3
  Demux1/4 -> Mux3/4
  Mux3/1 -> q_out/1
  Step size/1 -> Mux2/10
  q0/1 -> Mux2/9
  Clock/1 -> Mux2/8
  N_mt/1 -> Mux2/7
  h_mw/1 -> Mux2/6
  b(I)/1 -> Mux2/5
  R_sun(I)/1 -> Mux2/4
  Mux2/1 -> EKF/1
  EKF/1 -> Demux1/1
  Demux1/5 -> Mux4/1
  Demux1/6 -> Mux4/2
  Demux1/7 -> Mux4/3
  R_sun(S)/1 -> Mux2/1
  b(S)/1 -> Mux2/2
  Mux4/1 -> w_out/1

== system aausat3_lib/ADS/EKF using sun and mag vectors (AAUSAT3) ==
  Sun_S : Inport
  Mag_S : Inport  Port=2
  Omega_S : Inport  Port=3
  Sun_I : Inport  Port=4
  Mag_I : Inport  Port=5
  N_control : Inport  Port=6
  q0 : Inport  Port=7
  Eclipse : Inport  Port=8
  Clock : Clock
  Demux1 : Demux  Outputs=7
  EKF : MATLABFcn  MATLABFcn=EKFsimple  OutputDimensions=7  SampleTime=1
  Mux2 : Mux  Inputs=10
  Mux3 : Mux
  Mux4 : Mux  Inputs=3
  Step size : Constant
  q_out : Outport
  w_out : Outport  Port=2
  wires:
  Mux4/1 -> w_out/1
  Mag_S/1 -> Mux2/2
  Sun_S/1 -> Mux2/1
  Demux1/7 -> Mux4/3
  Demux1/6 -> Mux4/2
  Demux1/5 -> Mux4/1
  EKF/1 -> Demux1/1
  Mux2/1 -> EKF/1
  Sun_I/1 -> Mux2/4
  Mag_I/1 -> Mux2/5
  Mux3/1 -> q_out/1
  Demux1/4 -> Mux3/4
  Demux1/3 -> Mux3/3
  Demux1/2 -> Mux3/2
  Demux1/1 -> Mux3/1
  Omega_S/1 -> Mux2/3
  N_control/1 -> Mux2/6
  Clock/1 -> Mux2/7
  q0/1 -> Mux2/8
  Step size/1 -> Mux2/9
  Eclipse/1 -> Mux2/10

== system aausat3_lib/ADS/EKF using sun and mag vectors ..  and removing bias (AAUSAT-II) ==
  R_sun(S) : Inport
  b(S) : Inport  Port=2
  w(S) : Inport  Port=3
  R_sun(I) : Inport  Port=4
  b(I) : Inport  Port=5
  h_mw : Inport  Port=6
  N_mt : Inport  Port=7
  q0 : Inport  Port=8
  Eclipse : Inport  Port=9
  Clock : Clock
  EKF : MATLABFcn  MATLABFcn=AAUSAT_II_Kalman_BS_bias_vectors  OutputDimensions=7+12+12  SampleTime=0.1
  Mux2 : Mux  Inputs=11
  Selector : Selector  InputPortWidth=7+12+12  Indices=(1:4)
  Selector1 : Selector  InputPortWidth=7+12+12  Indices=(5:7)
  Selector2 : Selector  InputPortWidth=7+12+12  Indices=(8:19)
  Selector3 : Selector  InputPortWidth=7+12+12  Indices=(20:31)
  Step size : Constant  Value=0.1
  q_out : Outport
  w_out : Outport  Port=2
  residual : Outport  Port=3
  bias estimat : Outport  Port=4
  wires:
  Selector3/1 -> bias estimat/1
  Selector2/1 -> residual/1
  Selector1/1 -> w_out/1
  EKF/1 -> Selector3/1, Selector1/1, Selector2/1, Selector/1
  w(S)/1 -> Mux2/3
  Eclipse/1 -> Mux2/11
  Selector/1 -> q_out/1
  Step size/1 -> Mux2/10
  q0/1 -> Mux2/9
  Clock/1 -> Mux2/8
  N_mt/1 -> Mux2/7
  h_mw/1 -> Mux2/6
  b(I)/1 -> Mux2/5
  R_sun(I)/1 -> Mux2/4
  Mux2/1 -> EKF/1
  R_sun(S)/1 -> Mux2/1
  b(S)/1 -> Mux2/2

== system aausat3_lib/ADS/Propagator from Kalman filter (AAUSAT-II) ==
  q(S) : Inport
  w(S) : Inport  Port=2
  h_mw(S) : Inport  Port=3
  N_mt(S) : Inport  Port=4
  N_dist(S) : Inport  Port=5
  Inertia matrix : Inport  Port=6
  EKF : MATLABFcn  MATLABFcn=kalman-propagator  OutputDimensions=10  SampleTime=1
  Mux2 : Mux  Inputs=7
  Selector : Selector  InputPortWidth=10  Indices=(1:4)
  Selector1 : Selector  InputPortWidth=10  Indices=(5:7)
  Selector2 : Selector  InputPortWidth=10  Indices=(8:10)
  Step size : Constant
  q_out : Outport
  w_out : Outport  Port=2
  h_mw : Outport  Port=3
  wires:
  w(S)/1 -> Mux2/2
  q(S)/1 -> Mux2/1
  Mux2/1 -> EKF/1
  N_dist(S)/1 -> Mux2/5
  Step size/1 -> Mux2/6
  Selector/1 -> q_out/1
  h_mw(S)/1 -> Mux2/3
  EKF/1 -> Selector/1, Selector2/1, Selector1/1
  Selector1/1 -> w_out/1
  Selector2/1 -> h_mw/1
  N_mt(S)/1 -> Mux2/4
  Inertia matrix/1 -> Mux2/7

== system aausat3_lib/ADS/UKF using sun and mag vectors (AAUSAT3) ==
  Sun_S : Inport
  Mag_S : Inport  Port=2
  Omega_S : Inport  Port=3
  Sun_I : Inport  Port=4
  Mag_I : Inport  Port=5
  N_control : Inport  Port=6
  q0 : Inport  Port=7
  Eclipse : Inport  Port=8
  Enable : EnablePort
  Clock : Clock
  Demux1 : Demux  Outputs=7+9
  Mux1 : Mux  Inputs=9
  Mux2 : Mux  Inputs=10
  Mux3 : Mux
  Mux4 : Mux  Inputs=3
  Step size : Constant  Value=1/f_sample
  UKF : MATLABFcn  MATLABFcn=UKFsimple  OutputDimensions=7+9  SampleTime=1/f_sample
  q_out : Outport
  w_out : Outport  Port=2
  residual : Outport  Port=3
  wires:
  Mux1/1 -> residual/1
  Demux1/16 -> Mux1/9
  Demux1/15 -> Mux1/8
  Demux1/14 -> Mux1/7
  Demux1/13 -> Mux1/6
  Demux1/12 -> Mux1/5
  Demux1/11 -> Mux1/4
  Demux1/10 -> Mux1/3
  Demux1/9 -> Mux1/2
  Demux1/8 -> Mux1/1
  Eclipse/1 -> Mux2/10
  Step size/1 -> Mux2/9
  q0/1 -> Mux2/8
  Clock/1 -> Mux2/7
  N_control/1 -> Mux2/6
  Omega_S/1 -> Mux2/3
  Demux1/1 -> Mux3/1
  Demux1/2 -> Mux3/2
  Demux1/3 -> Mux3/3
  Demux1/4 -> Mux3/4
  Mux3/1 -> q_out/1
  Mag_I/1 -> Mux2/5
  Sun_I/1 -> Mux2/4
  Mux2/1 -> UKF/1
  UKF/1 -> Demux1/1
  Demux1/5 -> Mux4/1
  Demux1/6 -> Mux4/2
  Demux1/7 -> Mux4/3
  Sun_S/1 -> Mux2/1
  Mag_S/1 -> Mux2/2
  Mux4/1 -> w_out/1

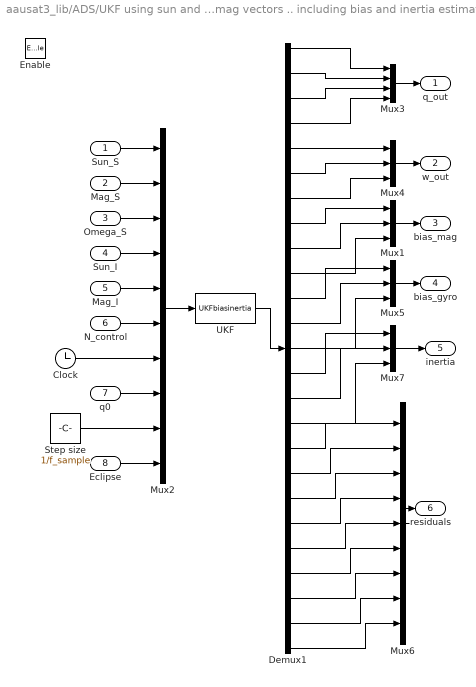
== system aausat3_lib/ADS/UKF using sun and mag vectors .. including bias and inertia estimation (AAUSAT3) ==
  Sun_S : Inport
  Mag_S : Inport  Port=2
  Omega_S : Inport  Port=3
  Sun_I : Inport  Port=4
  Mag_I : Inport  Port=5
  N_control : Inport  Port=6
  q0 : Inport  Port=7
  Eclipse : Inport  Port=8
  Enable : EnablePort
  Clock : Clock
  Demux1 : Demux  Outputs=25
  Mux{1,4..5,7} (4 alike) : Mux  Inputs=3
  Mux2 : Mux  Inputs=10
  Mux3 : Mux
  Mux6 : Mux  Inputs=9
  Step size : Constant  Value=1/f_sample
  UKF : MATLABFcn  MATLABFcn=UKFbiasinertia  OutputDimensions=25  SampleTime=1/f_sample
  q_out : Outport
  w_out : Outport  Port=2
  bias_mag : Outport  Port=3
  bias_gyro : Outport  Port=4
  inertia : Outport  Port=5
  residuals : Outport  Port=6
  wires:
  Eclipse/1 -> Mux2/10
  Step size/1 -> Mux2/9
  q0/1 -> Mux2/8
  Clock/1 -> Mux2/7
  N_control/1 -> Mux2/6
  Omega_S/1 -> Mux2/3
  Mux3/1 -> q_out/1
  Mag_I/1 -> Mux2/5
  Sun_I/1 -> Mux2/4
  Mux2/1 -> UKF/1
  UKF/1 -> Demux1/1
  Sun_S/1 -> Mux2/1
  Mag_S/1 -> Mux2/2
  Mux4/1 -> w_out/1
  Mux1/1 -> bias_mag/1
  Mux5/1 -> bias_gyro/1
  Mux6/1 -> residuals/1
  Mux7/1 -> inertia/1
  Demux1/1 -> Mux3/1
  Demux1/2 -> Mux3/2
  Demux1/3 -> Mux3/3
  Demux1/4 -> Mux3/4
  Demux1/5 -> Mux4/1
  Demux1/6 -> Mux4/2
  Demux1/7 -> Mux4/3
  Demux1/8 -> Mux1/1
  Demux1/9 -> Mux1/2
  Demux1/10 -> Mux1/3
  Demux1/11 -> Mux5/1
  Demux1/12 -> Mux5/2
  Demux1/13 -> Mux5/3
  Demux1/14 -> Mux7/1
  Demux1/15 -> Mux7/2
  Demux1/16 -> Mux7/3
  Demux1/17 -> Mux6/1
  Demux1/18 -> Mux6/2
  Demux1/19 -> Mux6/3
  Demux1/20 -> Mux6/4
  Demux1/21 -> Mux6/5
  Demux1/22 -> Mux6/6
  Demux1/23 -> Mux6/7
  Demux1/24 -> Mux6/8
  Demux1/25 -> Mux6/9

== system aausat3_lib/ADS/UKF using sun and mag vectors .. including bias estimation (AAUSAT3) ==
  Sun_S : Inport
  Mag_S : Inport  Port=2
  Omega_S : Inport  Port=3
  Sun_I : Inport  Port=4
  Mag_I : Inport  Port=5
  N_control : Inport  Port=6
  q0 : Inport  Port=7
  Eclipse : Inport  Port=8
  Enable : EnablePort
  Clock : Clock
  Demux1 : Demux  Outputs=22
  Mux1 : Mux  Inputs=3
  Mux2 : Mux  Inputs=10
  Mux3 : Mux
  Mux4 : Mux  Inputs=3
  Mux5 : Mux  Inputs=3
  Mux6 : Mux  Inputs=9
  Step size : Constant  Value=1/f_sample
  UKF : MATLABFcn  MATLABFcn=UKFbias  OutputDimensions=22  SampleTime=1/f_sample
  q_out : Outport
  w_out : Outport  Port=2
  bias_mag : Outport  Port=3
  bias_gyro : Outport  Port=4
  residuals : Outport  Port=5
  wires:
  Demux1/22 -> Mux6/9
  Demux1/21 -> Mux6/8
  Demux1/20 -> Mux6/7
  Demux1/19 -> Mux6/6
  Demux1/18 -> Mux6/5
  Demux1/17 -> Mux6/4
  Demux1/16 -> Mux6/3
  Demux1/15 -> Mux6/2
  Demux1/14 -> Mux6/1
  Demux1/13 -> Mux5/3
  Demux1/12 -> Mux5/2
  Demux1/11 -> Mux5/1
  Demux1/10 -> Mux1/3
  Demux1/9 -> Mux1/2
  Demux1/8 -> Mux1/1
  Demux1/7 -> Mux4/3
  Demux1/6 -> Mux4/2
  Demux1/5 -> Mux4/1
  Demux1/2 -> Mux3/2
  Demux1/4 -> Mux3/4
  Demux1/3 -> Mux3/3
  Demux1/1 -> Mux3/1
  Mux6/1 -> residuals/1
  Mux5/1 -> bias_gyro/1
  Mux1/1 -> bias_mag/1
  Mux4/1 -> w_out/1
  Mag_S/1 -> Mux2/2
  Sun_S/1 -> Mux2/1
  UKF/1 -> Demux1/1
  Mux2/1 -> UKF/1
  Sun_I/1 -> Mux2/4
  Mag_I/1 -> Mux2/5
  Mux3/1 -> q_out/1
  Omega_S/1 -> Mux2/3
  N_control/1 -> Mux2/6
  Clock/1 -> Mux2/7
  q0/1 -> Mux2/8
  Step size/1 -> Mux2/9
  Eclipse/1 -> Mux2/10

== system aausat3_lib/ADS/otoquest (AAUSAT-II) ==
  B (I) : Inport  SampleTime=1
  R_sun(I) : Inport  Port=2  SampleTime=1
  B(S) : Inport  Port=3  SampleTime=1
  R_sun(S) : Inport  Port=4  SampleTime=1
  Mux : Mux  Inputs=6
  Weights : Constant  Value=[0.5,0.5]
  create q_old : UnitDelay  InitialCondition=[0.8 0 0 0.6]
  otoquest.m : MATLABFcn  MATLABFcn=otoquest(u)  Output1D=off
  q(I->S) : Outport  PortDimensions=4
  wires:
  create q_old/1 -> Mux/6
  Mux/1 -> otoquest.m/1
  otoquest.m/1 -> create q_old/1, q(I->S)/1
  B (I)/1 -> Mux/1
  R_sun(I)/1 -> Mux/2
  B(S)/1 -> Mux/3
  R_sun(S)/1 -> Mux/4
  Weights/1 -> Mux/5

== system aausat3_lib/ADS/otoquest with propagator (AAUSAT-II) ==
  B (I) : Inport  SampleTime=1
  R_sun(I) : Inport  Port=2  SampleTime=1
  B(S) : Inport  Port=3  SampleTime=1
  R_sun(S) : Inport  Port=4  SampleTime=1
  omega : Inport  Port=5  SampleTime=1
  eclipse : Inport  Port=6  SampleTime=1
  Mux : Mux  Inputs=7
  Weights : Constant  Value=[0.5,0.5]
  otoquest.m : MATLABFcn  MATLABFcn=otoquest_with_pro(u)  Output1D=off  SampleTime=0.1
  q_p(I->S) : Outport  PortDimensions=4
  wires:
  Mux/1 -> otoquest.m/1
  otoquest.m/1 -> q_p(I->S)/1
  B (I)/1 -> Mux/1
  R_sun(I)/1 -> Mux/2
  B(S)/1 -> Mux/3
  R_sun(S)/1 -> Mux/4
  Weights/1 -> Mux/5
  eclipse/1 -> Mux/7
  omega/1 -> Mux/6

== system aausat3_lib/ADS/q-method (AAUSAT-II) ==
  q(E->I) : Inport  SampleTime=1
  R_s(I) : Inport  Port=2  SampleTime=1
  B(E) : Inport  Port=3  SampleTime=1
  B(sc) : Inport  Port=4  SampleTime=1
  R_s(sc) : Inport  Port=5  SampleTime=1
  Mux : Mux  Inputs=6
  To unit vector{,1..3} (4 alike) : aausat3_lib/Math Utilities/Vector operations/To unit vector  SystemSampleTime=-1
  Unit Delay : UnitDelay
  Vector rotation by q : aausat3_lib/Math Utilities/Quaternion operations/Vector rotation by q  SystemSampleTime=-1
  Weights : Constant  Value=[1,0]
  qmethod.m : MATLABFcn  MATLABFcn=qmethod([u(1) u(4);u(2) u(5);u(3) u(6)] , [u(7) u(10);u(8) u(11); u(9) u(12)], [u(13);u(14)],[u(15);u(16);u(17);u(18)])  Output1D=off
  q(I-SC) : Outport  PortDimensions=4
  wires:
  Weights/1 -> Mux/5
  Unit Delay/1 -> Mux/6
  R_s(sc)/1 -> To unit vector1/1
  To unit vector1/1 -> Mux/2
  To unit vector3/1 -> Mux/4
  R_s(I)/1 -> To unit vector3/1
  B(sc)/1 -> To unit vector/1
  Vector rotation by q/1 -> To unit vector2/1
  To unit vector2/1 -> Mux/3
  To unit vector/1 -> Mux/1
  Mux/1 -> qmethod.m/1
  B(E)/1 -> Vector rotation by q/2
  q(E->I)/1 -> Vector rotation by q/1
  qmethod.m/1 -> Unit Delay/1, q(I-SC)/1
